simulink model "fft_and_filter"  (R2015b)
settings: Solver=VariableStepAuto  StartTime=0.0  StopTime=1  MaxStep=1e-4  RelTol=1e-3
libraries: dspsrcs4 x1
settings Model: Creator=yehuohanxing  LastModifiedBy=yehuohanxing

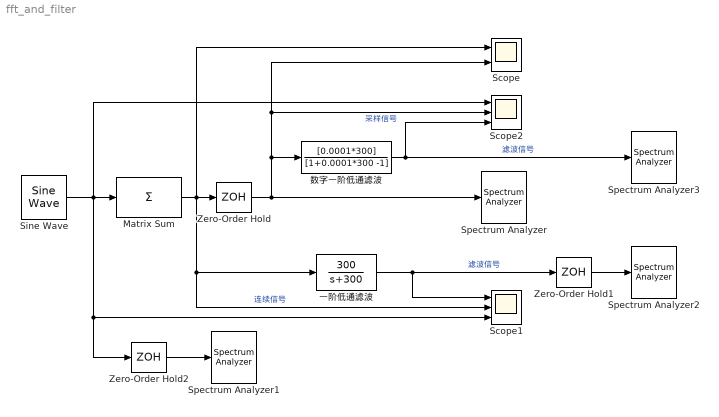
== system fft_and_filter ==
  Matrix Sum : Sum  Inputs=+  CollapseDim=2  OutDataTypeStr=Inherit: Same as first input
  Scope : Scope  NumInputPorts=2
  Scope1 : Scope  NumInputPorts=3
  Scope2 : Scope  NumInputPorts=3
  Sine Wave : dspsrcs4/Sine Wave  Amplitude=[3 1]  Frequency=[150 1000]  Phase=0  SampleMode=Continuous  OutComplex=Real  CompMethod=Trigonometric fcn  TableSize=Speed  SampleTime=1e-5  SamplesPerFrame=5  ResetState=Restart at time zero  OutputFrames=off  dataType=double  wordLen=16  udDataType=sfix(16)  fracBitsMode=Best precision  numFracBits=15  OutDataTypeStr=double  LastOutDataTypeStr=double
  Spectrum Analyzer{,1..3} (4 alike) : SpectrumAnalyzer
  Zero-Order Hold : ZeroOrderHold  SampleTime=0.0001
  Zero-Order Hold1 : ZeroOrderHold  SampleTime=0.0001
  Zero-Order Hold2 : ZeroOrderHold  SampleTime=0.0001
  一阶低通滤波 : TransferFcn  Numerator=[300]  Denominator=[1 300]
  数字一阶低通滤波 : DiscreteFilter  Numerator=[0.0001*300]  Denominator=[1+0.0001*300 -1]
  wires:
  Matrix Sum/1 -> Scope1/2, 一阶低通滤波/1, Scope/1, Zero-Order Hold/1  "连续信号"
  Zero-Order Hold/1 -> Spectrum Analyzer/1, 数字一阶低通滤波/1, Scope/2, Scope2/2  "采样信号"
  一阶低通滤波/1 -> Zero-Order Hold1/1, Scope1/1  "滤波信号"
  数字一阶低通滤波/1 -> Spectrum Analyzer3/1, Scope2/3  "滤波信号"
  Zero-Order Hold1/1 -> Spectrum Analyzer2/1
  Sine Wave/1 -> Scope2/1, Zero-Order Hold2/1, Scope1/3, Matrix Sum/1
  Zero-Order Hold2/1 -> Spectrum Analyzer1/1
